simulink model "time"  (R2017b)
settings: Solver=FixedStepAuto  StartTime=0.0  StopTime=10.0  FixedStep=1  RelTol=1e-3
undefined symbols (not defined in the file): DiscIntNeverNeededParam
libraries: GPIO_Lib x6, TIMERS_Lib x3, USART_Lib x3, simulink x1
(part 1 of 2)
settings Model: Creator=edupc  LastModifiedBy=edupc

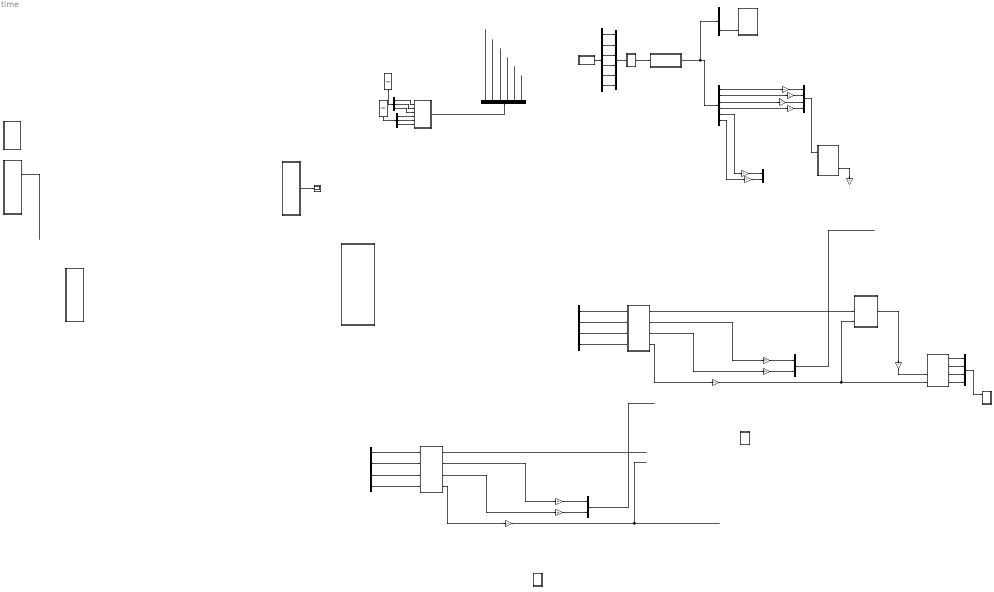
== system time ==
  Attitude : Subsystem  TreatAsAtomicUnit=on  SystemSampleTime=0.002
  Bus Creator : BusCreator  Inputs=6
  Bus Creator1 : BusCreator  Inputs=4
  Bus Creator2 : BusCreator  Inputs=2
  Bus Selector : BusSelector  OutputSignals=roll,pitch,yaw
  Bus Selector1 : BusSelector  OutputSignals=p,q,roll,pitch,yaw,r
  Chart : Stateflow chart  TreatAsAtomicUnit=on
  Chart1 : Stateflow chart  TreatAsAtomicUnit=on
  Chart2 : Stateflow chart  TreatAsAtomicUnit=on
  Chart3 : Stateflow chart  TreatAsAtomicUnit=on
  Chart4 : Stateflow chart  Priority=1  TreatAsAtomicUnit=on
  Chart9 : Stateflow chart  TreatAsAtomicUnit=on
  Data Type Conversion : DataTypeConversion  OutDataTypeStr=int32
  Data Type Conversion3 : DataTypeConversion  OutDataTypeStr=int32
  Demux1 : Demux
  Demux2 : Demux  Outputs=6
  Demux3 : Demux
  Demux4 : Demux  Outputs=3
  Demux5 : Demux  Outputs=3
  Demux6 : Demux  Outputs=6
  Filter : Subsystem  Tag=FilterWizardSubSystem  TreatAsAtomicUnit=on  SystemSampleTime=0.002
      settings: ErrorFcn=dspFilterRealizedInBasicElemsAlgLoopErrFcnCallback
  Gain{,1..2,11..13} (6 alike) : Gain  Gain=180/pi
  Gain10 : Gain  Gain=0.4
  Gain3 : Gain  Gain=30  ParamDataTypeStr=single
  Gain4 : Gain  Gain=30
  Gain5 : Gain  Gain=0.4
  Gain6 : Gain  Gain=-1  ParamDataTypeStr=single  OutDataTypeStr=single
  Gain7 : Gain  Gain=-1  ParamDataTypeStr=single  OutDataTypeStr=single
  Gain8 : Gain  Gain=30  ParamDataTypeStr=single
  Gain9 : Gain  Gain=30
  Mux1 : Mux  Inputs=2
  Mux2 : Mux
  Mux3 : Mux  Inputs=2
  PWM : Subsystem  TreatAsAtomicUnit=on
  Scope : Scope
  State Estimation and Complimentary Mixing : Subsystem  mask{EAComp=0.95}
      mask prompts: EAComp "Complimentary Filter Alpha:"
      mask TypeOptions EAComp: Complimentary Filter/EAComp
  Subsystem : Subsystem  TreatAsAtomicUnit=on  SystemSampleTime=0.002
  Subsystem1 : Subsystem  TreatAsAtomicUnit=on
  Subsystem5 : Subsystem  TreatAsAtomicUnit=on
  Yaw : Subsystem  TreatAsAtomicUnit=on  SystemSampleTime=0.002
  data scaling : Subsystem
  judgeLock : Subsystem  TreatAsAtomicUnit=on
  judgeLock1 : Subsystem  TreatAsAtomicUnit=on
  pwm_out1 : MATLAB Function  TreatAsAtomicUnit=on  SystemSampleTime=0.002
  wires:
  Chart/1(y) -> Scope/1
  Mux2/1 -> PWM/1(In1)
  Yaw/1(tau_yaw) -> Gain7/1
  Gain4/1 -> Mux1/2
  ? -> Yaw/1(states_estim)
  Gain5/1 -> Yaw/3(thrLow), pwm_out1/4(Thrust)
  Demux3/2 -> Subsystem5/2(pitchIn)
  Subsystem5/1(yaw) -> Yaw/2(yaw_ref)
  Subsystem5/4(thr) -> Gain5/1
  ? -> pwm_out1/2(Pitch)
  ? -> pwm_out1/1(Roll)
  Subsystem5/3(roll) -> Gain4/1
  pwm_out1/1(M1) -> Mux2/1
  Demux3/4 -> Subsystem5/4(yawIn)
  pwm_out1/3(M3) -> Mux2/3
  Demux3/3 -> Subsystem5/3(thrIn)
  Demux3/1 -> Subsystem5/1(rollIn)
  pwm_out1/2(M2) -> Mux2/2
  ? -> PWM/2(flyOk), judgeLock/1(In1)
  Subsystem5/2(pitch) -> Gain3/1
  Gain3/1 -> Mux1/1
  pwm_out1/4(M4) -> Mux2/4
  ? -> Demux3/1
  Gain7/1 -> pwm_out1/3(Yaw)
  Mux1/1 -> ?  "pitchRollCommand"
  Attitude/2(tau_pitch) -> Gain6/1
  Demux2/2 -> Bus Creator/2  "gy_filt"
  Bus Creator1/1 -> Attitude/1(states_estim)  "pitchRollBus"
  Bus Selector1/6 -> Gain13/1  "<r>"
  Bus Creator/1 -> data scaling/1(In1)
  Bus Selector1/2 -> Gain12/1  "<q>"
  Filter/1(Output) -> Demux2/1
  Demux2/6 -> Bus Creator/6  "az_filt"
  Bus Selector1/3 -> Gain/1  "<roll>"
  Demux2/1 -> Bus Creator/1  "gx_filt"
  Gain1/1 -> Bus Creator1/4  "pitch"
  Demux2/3 -> Bus Creator/3  "gz_filt"
  Gain12/1 -> Bus Creator1/2  "q"
  Bus Selector/3 -> Subsystem/3(yaw)  "<yaw>"
  Gain13/1 -> Bus Creator2/2  "r"
  Gain/1 -> Bus Creator1/3  "roll"
  Demux2/5 -> Bus Creator/5  "ay_filt"
  data scaling/1(Out1) -> State Estimation and Complimentary Mixing/1(In1)
  Gain11/1 -> Bus Creator1/1  "p"
  Bus Selector1/1 -> Gain11/1  "<p>"
  Bus Selector1/5 -> Gain2/1  "<yaw>"
  Gain2/1 -> Bus Creator2/1  "yaw"
  State Estimation and Complimentary Mixing/1(State Estimations) -> Bus Selector/1, Bus Selector1/1
  Demux2/4 -> Bus Creator/4  "ax_filt"
  Bus Selector1/4 -> Gain1/1  "<pitch>"
  ? -> ?  "input"
  Chart3/1(gyroData) -> ?
  Demux6/4 -> ?
  Demux4/3 -> Chart1/6(gz)
  Data Type Conversion3/1 -> Demux4/1
  Data Type Conversion/1 -> Demux5/1
  Demux6/2 -> ?
  Demux5/2 -> Chart1/2(ay)
  Demux4/2 -> Chart1/5(gy)
  Chart1/1(offset) -> Demux6/1
  Demux5/3 -> Chart1/3(az)
  Demux6/3 -> ?
  Demux6/1 -> ?
  Demux6/5 -> ?
  Demux4/1 -> Chart1/4(gx)
  Demux6/6 -> ?
  Demux5/1 -> Chart1/1(ax)
  ? -> Data Type Conversion3/1
  Demux1/2 -> Subsystem1/2(pitchIn)
  Demux1/4 -> Subsystem1/4(yawIn)
  Gain10/1 -> ?
  Demux1/1 -> Subsystem1/1(rollIn)
  Subsystem1/3(roll) -> Gain9/1
  Subsystem1/1(yaw) -> ?
  Gain9/1 -> Mux3/2
  ? -> judgeLock1/1(In1)
  Gain8/1 -> Mux3/1
  Subsystem1/4(thr) -> Gain10/1
  Subsystem1/2(pitch) -> Gain8/1
  Demux1/3 -> Subsystem1/3(thrIn)
  Mux3/1 -> ?  "pitchRollCommand"
  ? -> Demux1/1

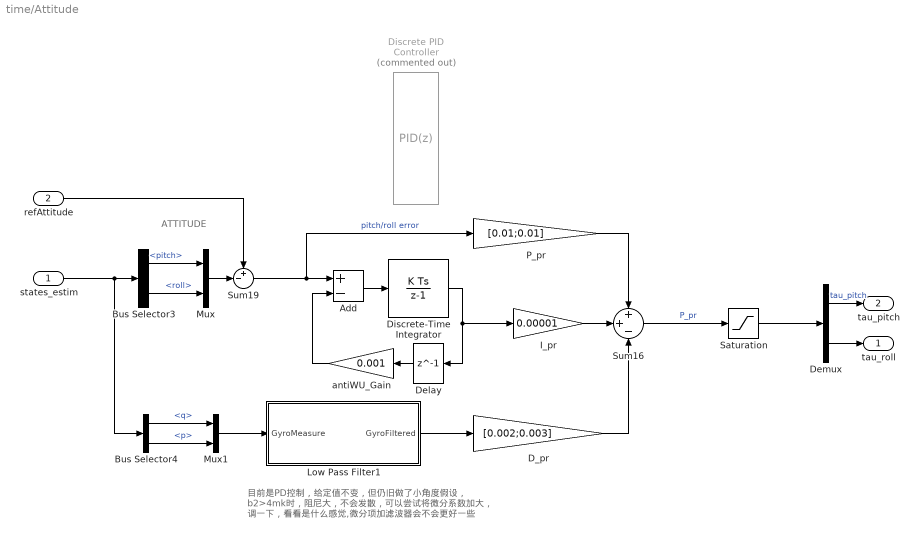
== system time/Attitude ==
  note: 目前是PD控制，给定值不变，但仍旧做了小角度假设，
      | b2>4mk时，阻尼大，不会发散，可以尝试将微分系数加大，
      | 调一下，看看是什么感觉,微分项加滤波器会不会更好一些
  note: ATTITUDE
  states_estim : Inport
  refAttitude : Inport  Port=2
  Add : Sum  Inputs=+-
  Bus Selector3 : BusSelector  OutputSignals=pitch,roll
  Bus Selector4 : BusSelector  OutputSignals=q,p
  D_pr : Gain  Gain=[0.002;0.003]  ParamDataTypeStr=single  OutDataTypeStr=single
  Delay : Delay  DelayLength=1  InitialCondition=0
  Demux : Demux  Outputs=2
  Discrete PID Controller : simulink/Continuous/PID Controller  Commented=on  Controller=PID  TimeDomain=Discrete-time  SampleTime=-1  IntegratorMethod=Forward Euler  FilterMethod=Forward Euler  Form=Parallel  UseFilter=on  ControllerParametersSource=external  P=1  I=1  D=0  N=100  InitialConditionSource=internal  InitialConditionForIntegrator=0  InitialConditionForFilter=0  ExternalReset=none  LimitOutput=off  UpperSaturationLimit=inf  LowerSaturationLimit=-inf  LinearizeAsGain=off  AntiWindupMode=none  Kb=1  TrackingMode=off  Kt=1  PParamMin=[]  PParamMax=[]  IParamMin=[]  IParamMax=[]  DParamMin=[]  DParamMax=[]  NParamMin=[]  NParamMax=[]  KbParamMin=[]  KbParamMax=[]  KtParamMin=[]  KtParamMax=[]  POutMin=[]  POutMax=[]  IOutMin=[]  IOutMax=[]  DOutMin=[]  DOutMax=[]  NOutMin=[]  NOutMax=[]  KbOutMin=[]  KbOutMax=[]  KtOutMin=[]  KtOutMax=[]  IntegratorOutMin=[]  IntegratorOutMax=[]  FilterOutMin=[]  FilterOutMax=[]  SumOutMin=[]  SumOutMax=[]  SumI1OutMin=[]  SumI1OutMax=[]  SumI2OutMin=[]  SumI2OutMax=[]  SumI3OutMin=[]  SumI3OutMax=[]  SumDOutMin=[]  SumDOutMax=[]  SaturationOutMin=[]  SaturationOutMax=[]  IntegratorContinuousStateAttributes=''  IntegratorStateMustResolveToSignalObject=off  IntegratorRTWStateStorageClass=Auto  FilterContinuousStateAttributes=''  FilterStateMustResolveToSignalObject=off  FilterRTWStateStorageClass=Auto  DifferentiatorICPrevScaledInput=0  DifferentiatorOutMin=[]  DifferentiatorOutMax=[]  InitialConditionSetting=State (most efficient)  FilterDiffOutCoefMin=[]  FilterDiffOutCoefMax=[]  SumDenOutMin=[]  SumDenOutMax=[]  SumNumOutMin=[]  SumNumOutMax=[]  ReciprocalOutMin=[]  ReciprocalOutMax=[]  DivideOutMin=[]  DivideOutMax=[]  TunerSelectOption=Transfer Function Based (PID Tuner App)
  Discrete-Time Integrator : DiscreteIntegrator  InitialConditionSetting=State (most efficient)  SampleTime=-1  LimitOutput=on  UpperSaturationLimit=0.1  LowerSaturationLimit=-0.1  ICPrevOutput=DiscIntNeverNeededParam  ICPrevScaledInput=DiscIntNeverNeededParam
  I_pr : Gain  Gain=0.00001  ParamDataTypeStr=single  OutDataTypeStr=single
  Low Pass Filter1 : Subsystem
  Mux : Mux  Inputs=2
  Mux1 : Mux  Inputs=2
  P_pr : Gain  Gain=[0.01;0.01]  ParamDataTypeStr=single  OutDataTypeStr=single
  Saturation : Saturate
  Sum16 : Sum  Inputs=++-  AccumDataTypeStr=single  OutDataTypeStr=single  SaturateOnIntegerOverflow=on
  Sum19 : Sum  Inputs=+-|
  antiWU_Gain : Gain  Gain=0.001
  tau_roll : Outport
  tau_pitch : Outport  Port=2
  wires:
  Mux1/1 -> Low Pass Filter1/1(GyroMeasure)
  Bus Selector4/2 -> Mux1/2  "<p>"
  Bus Selector3/2 -> Mux/2  "<roll>"
  Mux/1 -> Sum19/2
  refAttitude/1 -> Sum19/1
  states_estim/1 -> Bus Selector4/1, Bus Selector3/1
  D_pr/1 -> Sum16/3
  Demux/2 -> tau_roll/1
  Demux/1 -> tau_pitch/1  "tau_pitch"
  Delay/1 -> antiWU_Gain/1
  Discrete-Time Integrator/1 -> I_pr/1, Delay/1
  Sum19/1 -> P_pr/1, Add/1  "pitch/roll error"
  I_pr/1 -> Sum16/2
  P_pr/1 -> Sum16/1
  Bus Selector4/1 -> Mux1/1  "<q>"
  Bus Selector3/1 -> Mux/1  "<pitch>"
  Add/1 -> Discrete-Time Integrator/1
  antiWU_Gain/1 -> Add/2
  Sum16/1 -> Saturation/1  "P_pr"
  Saturation/1 -> Demux/1
  Low Pass Filter1/1(GyroFiltered) -> D_pr/1

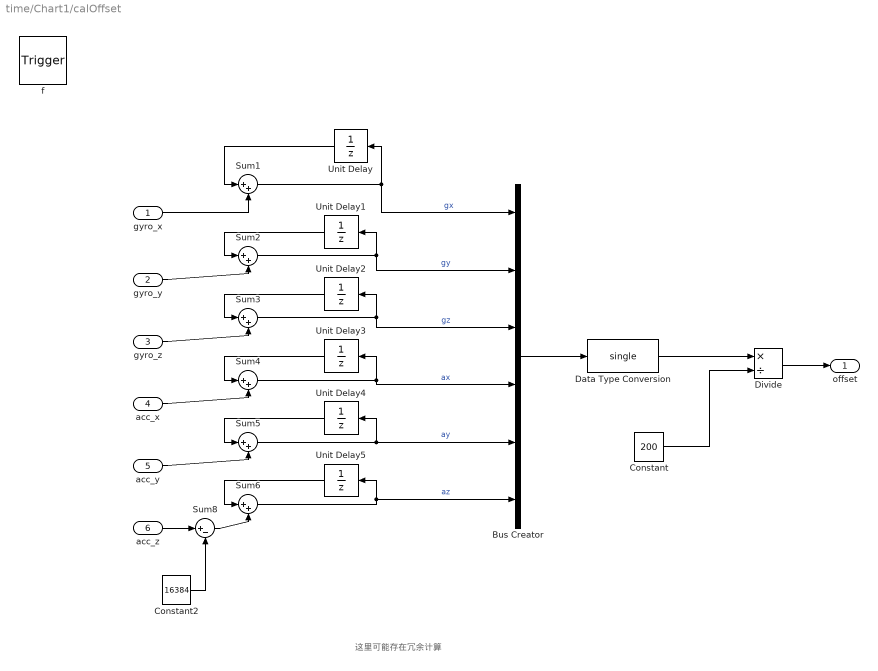
== system time/Chart1/calOffset ==
  note: 这里可能存在冗余计算
  gyro_x : Inport  OutDataTypeStr=int32
  gyro_y : Inport  Port=2  OutDataTypeStr=int32
  gyro_z : Inport  Port=3  OutDataTypeStr=int32
  acc_x : Inport  Port=4  OutDataTypeStr=int32
  acc_y : Inport  Port=5  OutDataTypeStr=int32
  acc_z : Inport  Port=6  OutDataTypeStr=int32
  f : TriggerPort  TriggerType=function-call  VariantControl=(inherit)
      settings: CopyFcn=Stateflow.SLINSF.SimulinkMan.removeBlockPreDeleteFcn  PreDeleteFcn=Stateflow.SLINSF.SimulinkMan.unsafePredeleteFcn
  Bus Creator : BusCreator  Inputs=6
  Constant : Constant  Value=200
  Constant2 : Constant  Value=16384  OutDataTypeStr=int16  SampleTime=-1
  Data Type Conversion : DataTypeConversion  OutDataTypeStr=single
  Divide : Product  Inputs=*/  OutDataTypeStr=single
  Sum{1..6} (6 alike) : Sum  Inputs=|++
  Sum8 : Sum  Inputs=|+-
  Unit Delay{,1..5} (6 alike) : UnitDelay  SampleTime=-1
  offset : Outport  OutDataTypeStr=single
  wires:
  gyro_x/1 -> Sum1/2
  Sum1/1 -> Bus Creator/1, Unit Delay/1  "gx"
  Unit Delay/1 -> Sum1/1
  gyro_y/1 -> Sum2/2
  Sum2/1 -> Unit Delay1/1, Bus Creator/2  "gy"
  Unit Delay1/1 -> Sum2/1
  Unit Delay2/1 -> Sum3/1
  Sum3/1 -> Unit Delay2/1, Bus Creator/3  "gz"
  Sum4/1 -> Unit Delay3/1, Bus Creator/4  "ax"
  Unit Delay3/1 -> Sum4/1
  Unit Delay4/1 -> Sum5/1
  Sum5/1 -> Unit Delay4/1, Bus Creator/5  "ay"
  Sum6/1 -> Bus Creator/6, Unit Delay5/1  "az"
  Unit Delay5/1 -> Sum6/1
  gyro_z/1 -> Sum3/2
  acc_x/1 -> Sum4/2
  acc_y/1 -> Sum5/2
  Bus Creator/1 -> Data Type Conversion/1
  acc_z/1 -> Sum8/1
  Sum8/1 -> Sum6/2
  Constant2/1 -> Sum8/2
  Constant/1 -> Divide/2
  Data Type Conversion/1 -> Divide/1
  Divide/1 -> offset/1

== system time/Chart4/pwmInit ==
  f : TriggerPort  TriggerType=function-call  VariantControl=(inherit)
      settings: CopyFcn=Stateflow.SLINSF.SimulinkMan.removeBlockPreDeleteFcn  PreDeleteFcn=Stateflow.SLINSF.SimulinkMan.unsafePredeleteFcn
  Constant : Constant
  Constant{10..13} (4 alike) : Constant  Value=0
  GPIO_Write : GPIO_Lib/GPIO_Write  Port_name=GPIOB  Pin0=off  Toggle_Pin0=off  Pin1=off  Toggle_Pin1=off  Pin2=on  Toggle_Pin2=off  Pin3=off  Toggle_Pin3=off  Pin4=off  Toggle_Pin4=off  Pin5=off  Toggle_Pin5=off  Pin6=off  Toggle_Pin6=off  Pin7=off  Toggle_Pin7=off  Pin8=off  Toggle_Pin8=off  Pin9=off  Toggle_Pin9=off  Pin10=off  Toggle_Pin10=off  Pin11=off  Toggle_Pin11=off  Pin12=off  Toggle_Pin12=off  Pin13=off  Toggle_Pin13=off  Pin14=off  Toggle_Pin14=off  Pin15=off  Toggle_Pin15=off  PinList="GPIOA4   8  11  12GPIOB1  2  3  6  7"
      settings: SourceProductName=Target Support Package - STM32 Adapter
  Timers : TIMERS_Lib/Timers  Priority=1  currentTIM=TIM2  TIM_Name=TIM2  TIM_APBClock=72000000  TIM_Set_Clk=on  TIM_Prescaler=71  TIM_Clock=1000000.00  Variable_frequency=off  TIM_Set_OutFreq=on  TIM_ARR=2500  Output_frequency=400.00  Repetition_counter=0  TIM_Mode=Up  TIM_DMA=none  TIM_IRQ=off  TIM_IRQ_ONLY=off  TIM_UP=off  TIM_TRG=off  TIM_COM=off  TIM_BRK=off  NbTIM=1  CH1_enable=on  CH1N_enable=off  CH1_type=Output_PWM  CH1_DMA=off  CH1_int=off  CH1_edge=Rising  CH1_div=1  CH1_variable_duty=on  CH1_set_pulse=off  CH1_output_duty=40.00  CH1_pulse=1000  CH2_enable=on  CH2N_enable=off  CH2_type=Output_PWM  CH2_DMA=off  CH2_int=off  CH2_edge=Rising  CH2_div=1  CH2_variable_duty=on  CH2_set_pulse=off  CH2_output_duty=40.00  CH2_pulse=1000  CH3_enable=on  CH3N_enable=off  CH3_type=Output_PWM  CH3_DMA=off  CH3_int=off  CH3_edge=Rising  CH3_div=1  CH3_variable_duty=on  CH3_set_pulse=off  CH3_output_duty=40.00  CH3_pulse=1000  CH4_enable=on  CH4N_enable=off  CH4_type=Output_PWM  CH4_DMA=off  CH4_int=off  CH4_edge=Rising  CH4_div=1  CH4_variable_duty=on  CH4_set_pulse=off  CH4_output_duty=40.00  CH4_pulse=1000
      settings: SourceProductName=Target Support Package - STM32 Adapter
  wires:
  Constant11/1 -> Timers/2
  Constant13/1 -> Timers/4
  Constant12/1 -> Timers/3
  Constant10/1 -> Timers/1
  Constant/1 -> GPIO_Write/1

== system time/Chart9/pwmInit ==
  f : TriggerPort  TriggerType=function-call  VariantControl=(inherit)
      settings: CopyFcn=Stateflow.SLINSF.SimulinkMan.removeBlockPreDeleteFcn  PreDeleteFcn=Stateflow.SLINSF.SimulinkMan.unsafePredeleteFcn
  Constant : Constant
  Constant{10..13} (4 alike) : Constant  Value=0
  GPIO_Write : GPIO_Lib/GPIO_Write  Port_name=GPIOB  Pin0=off  Toggle_Pin0=off  Pin1=off  Toggle_Pin1=off  Pin2=on  Toggle_Pin2=off  Pin3=off  Toggle_Pin3=off  Pin4=off  Toggle_Pin4=off  Pin5=off  Toggle_Pin5=off  Pin6=off  Toggle_Pin6=off  Pin7=off  Toggle_Pin7=off  Pin8=off  Toggle_Pin8=off  Pin9=off  Toggle_Pin9=off  Pin10=off  Toggle_Pin10=off  Pin11=off  Toggle_Pin11=off  Pin12=off  Toggle_Pin12=off  Pin13=off  Toggle_Pin13=off  Pin14=off  Toggle_Pin14=off  Pin15=off  Toggle_Pin15=off  PinList="GPIOA4   8  11  12GPIOB1  2  3  6  7"
      settings: SourceProductName=Target Support Package - STM32 Adapter
  Timers : TIMERS_Lib/Timers  Priority=1  currentTIM=TIM2  TIM_Name=TIM2  TIM_APBClock=72000000  TIM_Set_Clk=on  TIM_Prescaler=71  TIM_Clock=1000000.00  Variable_frequency=off  TIM_Set_OutFreq=on  TIM_ARR=2500  Output_frequency=400.00  Repetition_counter=0  TIM_Mode=Up  TIM_DMA=none  TIM_IRQ=off  TIM_IRQ_ONLY=off  TIM_UP=off  TIM_TRG=off  TIM_COM=off  TIM_BRK=off  NbTIM=1  CH1_enable=on  CH1N_enable=off  CH1_type=Output_PWM  CH1_DMA=off  CH1_int=off  CH1_edge=Rising  CH1_div=1  CH1_variable_duty=on  CH1_set_pulse=off  CH1_output_duty=40.00  CH1_pulse=1000  CH2_enable=on  CH2N_enable=off  CH2_type=Output_PWM  CH2_DMA=off  CH2_int=off  CH2_edge=Rising  CH2_div=1  CH2_variable_duty=on  CH2_set_pulse=off  CH2_output_duty=40.00  CH2_pulse=1000  CH3_enable=on  CH3N_enable=off  CH3_type=Output_PWM  CH3_DMA=off  CH3_int=off  CH3_edge=Rising  CH3_div=1  CH3_variable_duty=on  CH3_set_pulse=off  CH3_output_duty=40.00  CH3_pulse=1000  CH4_enable=on  CH4N_enable=off  CH4_type=Output_PWM  CH4_DMA=off  CH4_int=off  CH4_edge=Rising  CH4_div=1  CH4_variable_duty=on  CH4_set_pulse=off  CH4_output_duty=40.00  CH4_pulse=1000
      settings: SourceProductName=Target Support Package - STM32 Adapter
  wires:
  Constant11/1 -> Timers/2
  Constant13/1 -> Timers/4
  Constant12/1 -> Timers/3
  Constant10/1 -> Timers/1
  Constant/1 -> GPIO_Write/1

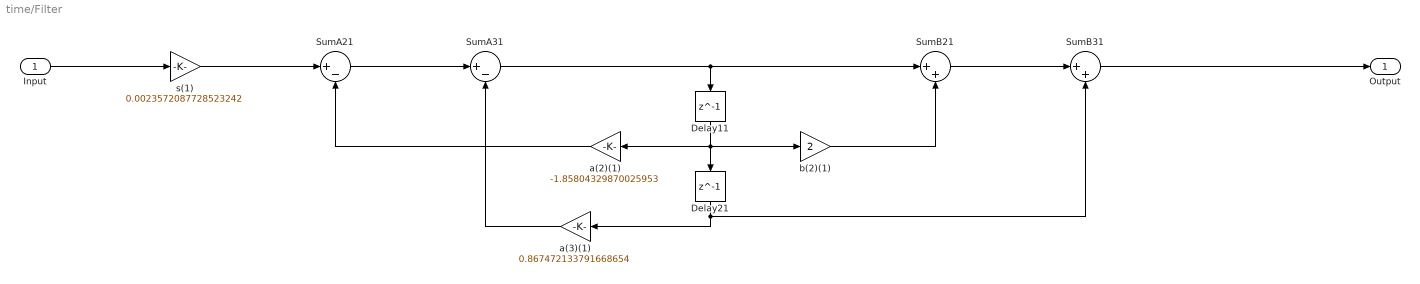
== system time/Filter ==
  Input : Inport
  Delay11 : Delay  DelayLength=1  InitialCondition=0
  Delay21 : Delay  DelayLength=1  InitialCondition=0
  SumA21 : Sum  Inputs=|+-  RndMeth=Nearest  SaturateOnIntegerOverflow=on  OutDataTypeStr=Inherit: Same as first input
  SumA31 : Sum  Inputs=|+-  RndMeth=Nearest  SaturateOnIntegerOverflow=on  OutDataTypeStr=Inherit: Same as first input
  SumB21 : Sum  Inputs=|++  RndMeth=Nearest  SaturateOnIntegerOverflow=on  OutDataTypeStr=Inherit: Same as first input
  SumB31 : Sum  Inputs=|++  RndMeth=Nearest  SaturateOnIntegerOverflow=on  OutDataTypeStr=Inherit: Same as first input
  a(2)(1) : Gain  Gain=-1.85804329870025953  ParamDataTypeStr=single  RndMeth=Nearest  SaturateOnIntegerOverflow=on  OutDataTypeStr=Inherit: Same as input
  a(3)(1) : Gain  Gain=0.867472133791668654  ParamDataTypeStr=single  RndMeth=Nearest  SaturateOnIntegerOverflow=on  OutDataTypeStr=Inherit: Same as input
  b(2)(1) : Gain  Gain=2  ParamDataTypeStr=single  RndMeth=Nearest  SaturateOnIntegerOverflow=on  OutDataTypeStr=Inherit: Same as input
  s(1) : Gain  Gain=0.0023572087728523242  ParamDataTypeStr=single  RndMeth=Nearest  SaturateOnIntegerOverflow=on  OutDataTypeStr=Inherit: Same as input
  Output : Outport
  wires:
  Input/1 -> s(1)/1
  s(1)/1 -> SumA21/1
  SumA21/1 -> SumA31/1
  SumA31/1 -> SumB21/1, Delay11/1
  SumB21/1 -> SumB31/1
  SumB31/1 -> Output/1
  a(2)(1)/1 -> SumA21/2
  Delay11/1 -> a(2)(1)/1, b(2)(1)/1, Delay21/1
  b(2)(1)/1 -> SumB21/2
  a(3)(1)/1 -> SumA31/2
  Delay21/1 -> a(3)(1)/1, SumB31/2

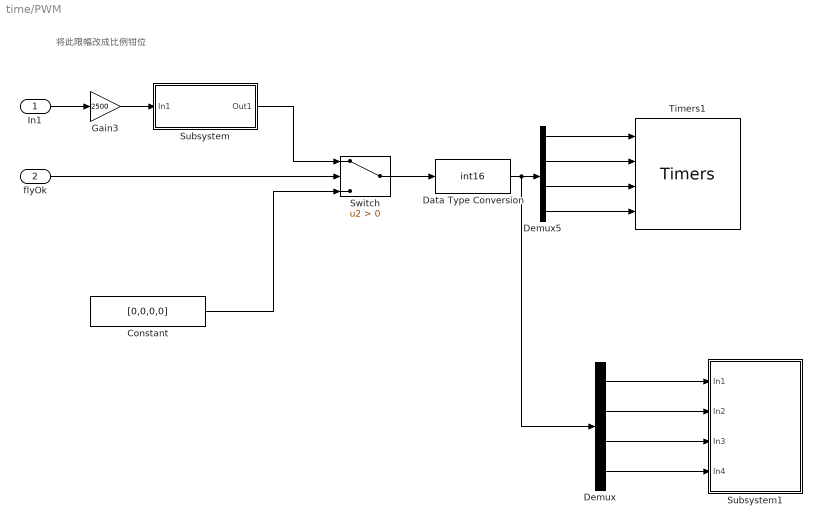
== system time/PWM ==
  note: 将此限幅改成比例钳位
  In1 : Inport
  flyOk : Inport  Port=2
  Constant : Constant  Value=[0,0,0,0]
  Data Type Conversion : DataTypeConversion  OutDataTypeStr=int16
  Demux : Demux
  Demux5 : Demux
  Gain3 : Gain  Gain=2500
  Subsystem : Subsystem
  Subsystem1 : Subsystem  TreatAsAtomicUnit=on
  Switch : Switch  Criteria=u2 > Threshold
  Timers1 : TIMERS_Lib/Timers  Priority=1  currentTIM=TIM2  TIM_Name=TIM2  TIM_APBClock=72000000  TIM_Set_Clk=on  TIM_Prescaler=71  TIM_Clock=1000000.00  Variable_frequency=off  TIM_Set_OutFreq=on  TIM_ARR=2500  Output_frequency=400.00  Repetition_counter=0  TIM_Mode=Up  TIM_DMA=none  TIM_IRQ=off  TIM_IRQ_ONLY=off  TIM_UP=off  TIM_TRG=off  TIM_COM=off  TIM_BRK=off  NbTIM=1  CH1_enable=on  CH1N_enable=off  CH1_type=Output_PWM  CH1_DMA=off  CH1_int=off  CH1_edge=Rising  CH1_div=1  CH1_variable_duty=on  CH1_set_pulse=off  CH1_output_duty=40.00  CH1_pulse=1000  CH2_enable=on  CH2N_enable=off  CH2_type=Output_PWM  CH2_DMA=off  CH2_int=off  CH2_edge=Rising  CH2_div=1  CH2_variable_duty=on  CH2_set_pulse=off  CH2_output_duty=40.00  CH2_pulse=1000  CH3_enable=on  CH3N_enable=off  CH3_type=Output_PWM  CH3_DMA=off  CH3_int=off  CH3_edge=Rising  CH3_div=1  CH3_variable_duty=on  CH3_set_pulse=off  CH3_output_duty=40.00  CH3_pulse=1000  CH4_enable=on  CH4N_enable=off  CH4_type=Output_PWM  CH4_DMA=off  CH4_int=off  CH4_edge=Rising  CH4_div=1  CH4_variable_duty=on  CH4_set_pulse=off  CH4_output_duty=40.00  CH4_pulse=1000
      settings: SourceProductName=Target Support Package - STM32 Adapter
  wires:
  Switch/1 -> Data Type Conversion/1
  Demux5/1 -> Timers1/1
  Demux5/4 -> Timers1/4
  Demux5/2 -> Timers1/2
  Demux5/3 -> Timers1/3
  flyOk/1 -> Switch/2
  Gain3/1 -> Subsystem/1(In1)
  In1/1 -> Gain3/1
  Data Type Conversion/1 -> Demux/1, Demux5/1
  Constant/1 -> Switch/3
  Subsystem/1(Out1) -> Switch/1
  Demux/1 -> Subsystem1/1(In1)
  Demux/2 -> Subsystem1/2(In2)
  Demux/3 -> Subsystem1/3(In3)
  Demux/4 -> Subsystem1/4(In4)

== system time/State Estimation and Complimentary Mixing ==
  note: The specific state estimation procedure employed in these bocks is
      | to be considered experimental (like everything else in this simulation).
      | While functional within the context of our application, this is not to be taken
      | as a "correct" method for state estimation or gyro/accelerometer data combination.
  note: Note:
      | x_gyro is taken as P,
      | y_gyro as Q,
      | z_gyro ad R.
  In1 : Inport
  Bus Creator : BusCreator  Inputs=6
  Bus Selector : BusSelector  OutputSignals=p,q,r,x_acc,y_acc,z_acc
  Complimentary Filter : Subsystem  mask{EAComp=EAComp}
      mask prompts: EAComp "Complimentary Filter Alpha:"
      mask TypeOptions EAComp: EAComp1/Gain
  Subsystem : Subsystem
  Subsystem1 : Subsystem
  State Estimations : Outport
  wires:
  In1/1 -> Bus Selector/1
  Bus Selector/1 -> Bus Creator/4, Subsystem/3(P)  "<p>"
  Bus Selector/3 -> Bus Creator/6, Subsystem/5(R)  "<r>"
  Bus Selector/2 -> Bus Creator/5, Subsystem/4(Q)  "<q>"
  Subsystem/2(thetaDot_gyro) -> Complimentary Filter/2(theDot_gyro)  "thateDot_gyro"
  Subsystem/3(psiDot_gyro) -> Complimentary Filter/3(psiDot_gyro)  "psiDot_gyro"
  Subsystem/1(phiDot_gyro) -> Complimentary Filter/1(phiDot_gyro)  "phiDot_gyro"
  Complimentary Filter/1(phi_est) -> Bus Creator/1, Subsystem/1(Phi)  "roll"
  Complimentary Filter/2(theta_est) -> Bus Creator/2, Subsystem/2(Theta)  "pitch"
  Complimentary Filter/3(psi_est) -> Bus Creator/3  "yaw"
  Subsystem1/2(phi_acc) -> Complimentary Filter/5(phiDot_acc)  "phi_acc"
  Subsystem1/1(theta_acc) -> Complimentary Filter/4(the_acc)  "theta_acc"
  Bus Selector/4 -> Subsystem1/1(x_acc)  "<x_acc>"
  Bus Selector/5 -> Subsystem1/2(y_acc)  "<y_acc>"
  Bus Selector/6 -> Subsystem1/3(z_acc)  "<z_acc>"
  Bus Creator/1 -> State Estimations/1

== system time/Subsystem ==
  roll : Inport
  pitch : Inport  Port=2
  yaw : Inport  Port=3
  Chart1 : Stateflow chart  TreatAsAtomicUnit=on
  wires:
  roll/1 -> Chart1/1(roll)
  yaw/1 -> Chart1/3(yaw)
  pitch/1 -> Chart1/2(pitch)

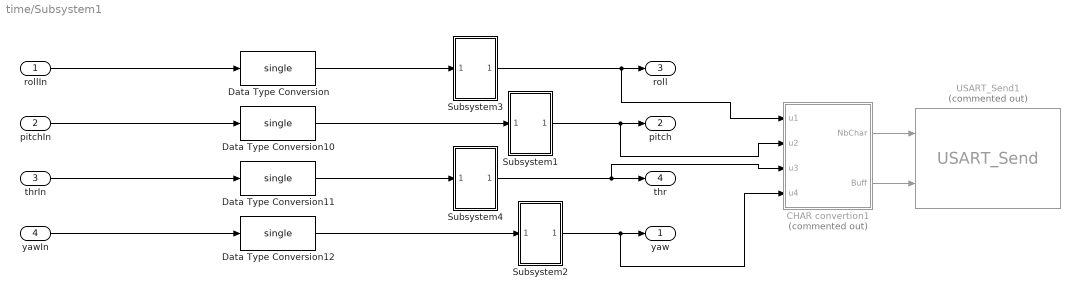
== system time/Subsystem1 ==
  rollIn : Inport
  pitchIn : Inport  Port=2
  thrIn : Inport  Port=3
  yawIn : Inport  Port=4
  CHAR convertion1 : MATLAB Function  Commented=on  TreatAsAtomicUnit=on
  Data Type Conversion{,10..12} (4 alike) : DataTypeConversion  OutDataTypeStr=single
  Subsystem1 : Subsystem
  Subsystem2 : Subsystem
  Subsystem3 : Subsystem
  Subsystem4 : Subsystem
  USART_Send1 : USART_Lib/USART_Send  Commented=on  USART_name=USART1  Buff_size=512  nbUsart=1  usartMode=Asynchronous  usartDma_Rx=off  usartDma_Tx=off  usartIt=on
      settings: SourceProductName=Target Support Package - STM32 Adapter
  yaw : Outport
  pitch : Outport  Port=2
  roll : Outport  Port=3
  thr : Outport  Port=4
  wires:
  Subsystem1/1(Out1) -> CHAR convertion1/2(u2), pitch/1
  Subsystem3/1(Out1) -> CHAR convertion1/1(u1), roll/1
  pitchIn/1 -> Data Type Conversion10/1
  yawIn/1 -> Data Type Conversion12/1
  rollIn/1 -> Data Type Conversion/1
  Data Type Conversion11/1 -> Subsystem4/1(In1)
  Data Type Conversion/1 -> Subsystem3/1(In1)
  Data Type Conversion12/1 -> Subsystem2/1(In1)
  Data Type Conversion10/1 -> Subsystem1/1(In1)
  thrIn/1 -> Data Type Conversion11/1
  Subsystem4/1(Out1) -> CHAR convertion1/3(u3), thr/1
  CHAR convertion1/2(Buff) -> USART_Send1/2
  CHAR convertion1/1(NbChar) -> USART_Send1/1
  Subsystem2/1(Out1) -> CHAR convertion1/4(u4), yaw/1

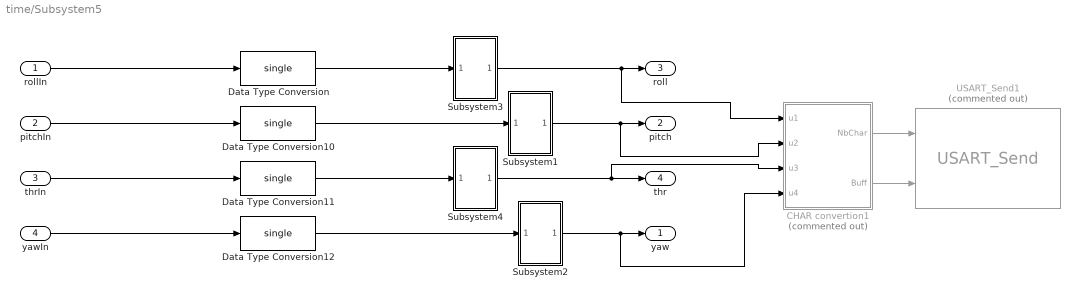
== system time/Subsystem5 ==
  rollIn : Inport
  pitchIn : Inport  Port=2
  thrIn : Inport  Port=3
  yawIn : Inport  Port=4
  CHAR convertion1 : MATLAB Function  Commented=on  TreatAsAtomicUnit=on
  Data Type Conversion{,10..12} (4 alike) : DataTypeConversion  OutDataTypeStr=single
  Subsystem1 : Subsystem
  Subsystem2 : Subsystem
  Subsystem3 : Subsystem
  Subsystem4 : Subsystem
  USART_Send1 : USART_Lib/USART_Send  Commented=on  USART_name=USART1  Buff_size=512  nbUsart=1  usartMode=Asynchronous  usartDma_Rx=off  usartDma_Tx=off  usartIt=on
      settings: SourceProductName=Target Support Package - STM32 Adapter
  yaw : Outport
  pitch : Outport  Port=2
  roll : Outport  Port=3
  thr : Outport  Port=4
  wires:
  Subsystem1/1(Out1) -> CHAR convertion1/2(u2), pitch/1
  Subsystem3/1(Out1) -> CHAR convertion1/1(u1), roll/1
  pitchIn/1 -> Data Type Conversion10/1
  yawIn/1 -> Data Type Conversion12/1
  rollIn/1 -> Data Type Conversion/1
  Data Type Conversion11/1 -> Subsystem4/1(In1)
  Data Type Conversion/1 -> Subsystem3/1(In1)
  Data Type Conversion12/1 -> Subsystem2/1(In1)
  Data Type Conversion10/1 -> Subsystem1/1(In1)
  thrIn/1 -> Data Type Conversion11/1
  Subsystem4/1(Out1) -> CHAR convertion1/3(u3), thr/1
  CHAR convertion1/2(Buff) -> USART_Send1/2
  CHAR convertion1/1(NbChar) -> USART_Send1/1
  Subsystem2/1(Out1) -> CHAR convertion1/4(u4), yaw/1

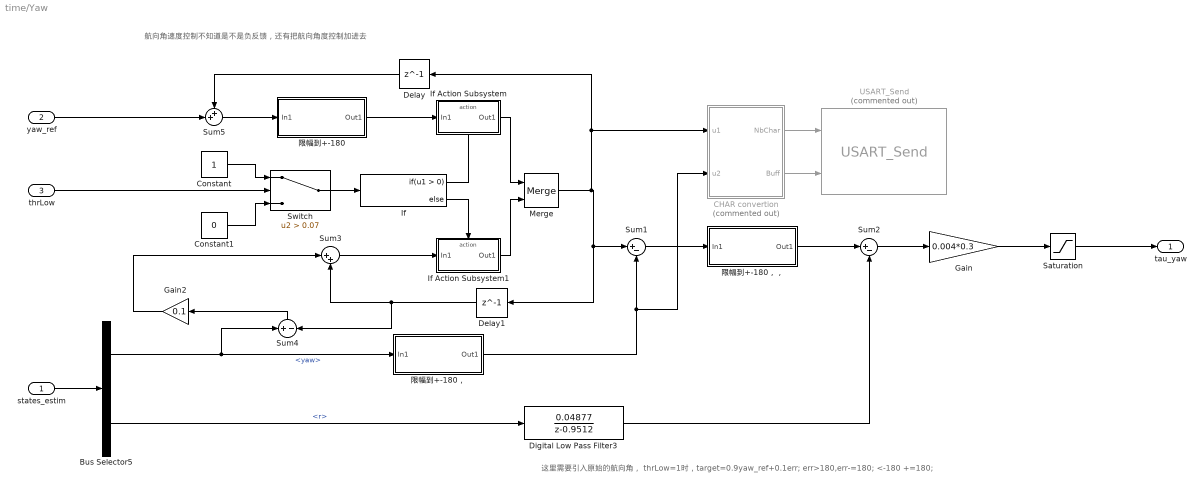
== system time/Yaw ==
  note: 这里需要引入原始的航向角，
      | thrLow=1时，target=0.9yaw_ref+0.1err;
      | err>180,err-=180;
      | <-180 +=180;
  note: 航向角速度控制不知道是不是负反馈，还有把航向角度控制加进去
  states_estim : Inport
  yaw_ref : Inport  Port=2
  thrLow : Inport  Port=3
  Bus Selector5 : BusSelector  OutputSignals=yaw,r
  CHAR convertion : MATLAB Function  Commented=on  TreatAsAtomicUnit=on
  Constant : Constant  OutDataTypeStr=int8
  Constant1 : Constant  Value=0  OutDataTypeStr=int8
  Delay : Delay  DelayLength=1
  Delay1 : Delay  DelayLength=1
  Digital Low Pass Filter3 : DiscreteTransferFcn  Numerator=[0.04877]  Denominator=[1 -0.9512]  OutDataTypeStr=int16
  Gain : Gain  Gain=0.004*0.3
  Gain2 : Gain  Gain=0.1
  If : If
  If Action Subsystem : Subsystem  TreatAsAtomicUnit=on
  If Action Subsystem1 : Subsystem  TreatAsAtomicUnit=on
  Merge : Merge
  Saturation : Saturate  UpperLimit=0.3  LowerLimit=-0.3
  Sum1 : Sum  Inputs=|+-
  Sum2 : Sum  Inputs=|+-
  Sum3 : Sum  Inputs=|++
  Sum4 : Sum  Inputs=+|-
  Sum5 : Sum  Inputs=++|
  Switch : Switch  Criteria=u2 > Threshold  Threshold=0.07
  USART_Send : USART_Lib/USART_Send  Commented=on  USART_name=USART1  Buff_size=512  nbUsart=1  usartMode=Asynchronous  usartDma_Rx=off  usartDma_Tx=off  usartIt=on
      settings: SourceProductName=Target Support Package - STM32 Adapter
  限幅到+-180 : Subsystem
  限幅到+-180， : Subsystem
  限幅到+-180，， : Subsystem
  tau_yaw : Outport
  wires:
  Gain/1 -> Saturation/1
  Sum2/1 -> Gain/1
  states_estim/1 -> Bus Selector5/1
  Bus Selector5/2 -> Digital Low Pass Filter3/1  "<r>"
  thrLow/1 -> Switch/2
  Constant/1 -> Switch/1
  Constant1/1 -> Switch/3
  Saturation/1 -> tau_yaw/1
  Switch/1 -> If/1
  If/1 -> If Action Subsystem/Action
  If Action Subsystem/1(Out1) -> Merge/1
  If/2 -> If Action Subsystem1/Action
  If Action Subsystem1/1(Out1) -> Merge/2
  Merge/1 -> CHAR convertion/1(u1), Delay/1, Delay1/1, Sum1/1
  Sum1/1 -> 限幅到+-180，，/1(In1)
  Bus Selector5/1 -> Sum4/1, 限幅到+-180，/1(In1)  "<yaw>"
  Sum3/1 -> If Action Subsystem1/1(In1)
  限幅到+-180/1(Out1) -> If Action Subsystem/1(In1)
  限幅到+-180，，/1(Out1) -> Sum2/1
  Sum5/1 -> 限幅到+-180/1(In1)
  yaw_ref/1 -> Sum5/2
  Delay/1 -> Sum5/1
  Delay1/1 -> Sum3/2, Sum4/2
  Sum4/1 -> Gain2/1
  Gain2/1 -> Sum3/1
  CHAR convertion/2(Buff) -> USART_Send/2
  CHAR convertion/1(NbChar) -> USART_Send/1
  限幅到+-180，/1(Out1) -> CHAR convertion/2(u2), Sum1/2
  Digital Low Pass Filter3/1 -> Sum2/2

== system time/data scaling ==
  note: For simulation, no
      | offset value is calculated.
  In1 : Inport
  Bus Creator : BusCreator  Inputs=6
  Bus Selector : BusSelector  OutputSignals=gx_filt,gy_filt,gz_filt,ax_filt,ay_filt,az_filt
  Demux : Demux  Outputs=3
  Demux1 : Demux  Outputs=3
  Gain : Gain  Gain=pi/(180*16.4)
  Gain1 : Gain  Gain=9.81/16384
  Mux1 : Mux  Inputs=3
  Mux2 : Mux  Inputs=3
  Out1 : Outport
  wires:
  In1/1 -> Bus Selector/1
  Bus Selector/1 -> Mux1/1  "<gx_filt>"
  Bus Selector/2 -> Mux1/2  "<gy_filt>"
  Bus Selector/3 -> Mux1/3  "<gz_filt>"
  Bus Selector/4 -> Mux2/1  "<ax_filt>"
  Bus Selector/5 -> Mux2/2  "<ay_filt>"
  Bus Selector/6 -> Mux2/3  "<az_filt>"
  Mux2/1 -> Gain1/1
  Mux1/1 -> Gain/1
  Gain1/1 -> Demux1/1
  Gain/1 -> Demux/1
  Demux/1 -> Bus Creator/1  "p"
  Demux/2 -> Bus Creator/2  "q"
  Demux/3 -> Bus Creator/3  "r"
  Demux1/1 -> Bus Creator/4  "x_acc"
  Demux1/2 -> Bus Creator/5  "y_acc"
  Demux1/3 -> Bus Creator/6  "z_acc"
  Bus Creator/1 -> Out1/1

== system time/judgeLock ==
  In1 : Inport
  Constant3 : Constant
  Constant4 : Constant  Value=0
  GPIO_Write : GPIO_Lib/GPIO_Write  Port_name=GPIOA  Pin0=off  Toggle_Pin0=off  Pin1=off  Toggle_Pin1=off  Pin2=off  Toggle_Pin2=off  Pin3=off  Toggle_Pin3=off  Pin4=off  Toggle_Pin4=off  Pin5=off  Toggle_Pin5=off  Pin6=off  Toggle_Pin6=off  Pin7=off  Toggle_Pin7=off  Pin8=on  Toggle_Pin8=off  Pin9=off  Toggle_Pin9=off  Pin10=off  Toggle_Pin10=off  Pin11=on  Toggle_Pin11=off  Pin12=off  Toggle_Pin12=off  Pin13=off  Toggle_Pin13=off  Pin14=off  Toggle_Pin14=off  Pin15=off  Toggle_Pin15=off  PinList="GPIOA4   8  11  12GPIOB1  2  3  6  7"
      settings: SourceProductName=Target Support Package - STM32 Adapter
  GPIO_Write1 : GPIO_Lib/GPIO_Write  Port_name=GPIOB  Pin0=off  Toggle_Pin0=off  Pin1=on  Toggle_Pin1=off  Pin2=off  Toggle_Pin2=off  Pin3=on  Toggle_Pin3=off  Pin4=off  Toggle_Pin4=off  Pin5=off  Toggle_Pin5=off  Pin6=off  Toggle_Pin6=off  Pin7=off  Toggle_Pin7=off  Pin8=off  Toggle_Pin8=off  Pin9=off  Toggle_Pin9=off  Pin10=off  Toggle_Pin10=off  Pin11=off  Toggle_Pin11=off  Pin12=off  Toggle_Pin12=off  Pin13=off  Toggle_Pin13=off  Pin14=off  Toggle_Pin14=off  Pin15=off  Toggle_Pin15=off  PinList="GPIOA4   8  11  12GPIOB1  2  3  6  7"
      settings: SourceProductName=Target Support Package - STM32 Adapter
  If : If
  If Action Subsystem : Subsystem  TreatAsAtomicUnit=on
  If Action Subsystem1 : Subsystem  TreatAsAtomicUnit=on
  Merge : Merge
  wires:
  In1/1 -> If/1
  Constant4/1 -> If Action Subsystem1/1(In1)
  Constant3/1 -> If Action Subsystem/1(In1)
  If Action Subsystem1/1(Out1) -> Merge/2
  If/1 -> If Action Subsystem/Action
  If/2 -> If Action Subsystem1/Action
  If Action Subsystem/1(Out1) -> Merge/1
  Merge/1 -> GPIO_Write/1, GPIO_Write/2, GPIO_Write1/2, GPIO_Write1/1

== system time/judgeLock1 ==
  In1 : Inport
  Constant3 : Constant
  Constant4 : Constant  Value=0
  GPIO_Write : GPIO_Lib/GPIO_Write  Port_name=GPIOA  Pin0=off  Toggle_Pin0=off  Pin1=off  Toggle_Pin1=off  Pin2=off  Toggle_Pin2=off  Pin3=off  Toggle_Pin3=off  Pin4=off  Toggle_Pin4=off  Pin5=off  Toggle_Pin5=off  Pin6=off  Toggle_Pin6=off  Pin7=off  Toggle_Pin7=off  Pin8=on  Toggle_Pin8=off  Pin9=off  Toggle_Pin9=off  Pin10=off  Toggle_Pin10=off  Pin11=on  Toggle_Pin11=off  Pin12=off  Toggle_Pin12=off  Pin13=off  Toggle_Pin13=off  Pin14=off  Toggle_Pin14=off  Pin15=off  Toggle_Pin15=off  PinList="GPIOA4   8  11  12GPIOB1  2  3  6  7"
      settings: SourceProductName=Target Support Package - STM32 Adapter
  GPIO_Write1 : GPIO_Lib/GPIO_Write  Port_name=GPIOB  Pin0=off  Toggle_Pin0=off  Pin1=on  Toggle_Pin1=off  Pin2=off  Toggle_Pin2=off  Pin3=on  Toggle_Pin3=off  Pin4=off  Toggle_Pin4=off  Pin5=off  Toggle_Pin5=off  Pin6=off  Toggle_Pin6=off  Pin7=off  Toggle_Pin7=off  Pin8=off  Toggle_Pin8=off  Pin9=off  Toggle_Pin9=off  Pin10=off  Toggle_Pin10=off  Pin11=off  Toggle_Pin11=off  Pin12=off  Toggle_Pin12=off  Pin13=off  Toggle_Pin13=off  Pin14=off  Toggle_Pin14=off  Pin15=off  Toggle_Pin15=off  PinList="GPIOA4   8  11  12GPIOB1  2  3  6  7"
      settings: SourceProductName=Target Support Package - STM32 Adapter
  If : If
  If Action Subsystem : Subsystem  TreatAsAtomicUnit=on
  If Action Subsystem1 : Subsystem  TreatAsAtomicUnit=on
  Merge : Merge
  wires:
  In1/1 -> If/1
  Constant4/1 -> If Action Subsystem1/1(In1)
  Constant3/1 -> If Action Subsystem/1(In1)
  If Action Subsystem1/1(Out1) -> Merge/2
  If/1 -> If Action Subsystem/Action
  If/2 -> If Action Subsystem1/Action
  If Action Subsystem/1(Out1) -> Merge/1
  Merge/1 -> GPIO_Write/1, GPIO_Write/2, GPIO_Write1/2, GPIO_Write1/1

== system time/Attitude/Low Pass Filter1 ==
  GyroMeasure : Inport
  Demux : Demux  Outputs=2
  Digital Low Pass Filter1 : DiscreteTransferFcn  Numerator=[0.04877]  Denominator=[1 -0.9512]  OutDataTypeStr=int16
  Digital Low Pass Filter2 : DiscreteTransferFcn  Numerator=[0.04877]  Denominator=[1 -0.9512]  OutDataTypeStr=int16
  Mux3 : Mux  Inputs=2
  GyroFiltered : Outport
  wires:
  Mux3/1 -> GyroFiltered/1
  Demux/1 -> Digital Low Pass Filter2/1
  GyroMeasure/1 -> Demux/1
  Demux/2 -> Digital Low Pass Filter1/1
  Digital Low Pass Filter2/1 -> Mux3/1
  Digital Low Pass Filter1/1 -> Mux3/2

== system time/PWM/Subsystem ==
  In1 : Inport
  Demux : Demux
  Divide : Product  Inputs=*/
  Gain : Gain  Gain=1200
  If : If  IfExpression=u1 > 1200
  If Action Subsystem : Subsystem  TreatAsAtomicUnit=on
  If Action Subsystem1 : Subsystem  TreatAsAtomicUnit=on
  Merge : Merge
  Min : MinMax  Function=max  Inputs=4
  Out1 : Outport
  wires:
  Demux/4 -> Min/4
  In1/1 -> Divide/1, If Action Subsystem1/1(In1), Demux/1
  Demux/1 -> Min/1
  Demux/2 -> Min/2
  Demux/3 -> Min/3
  If/1 -> If Action Subsystem/Action
  If/2 -> If Action Subsystem1/Action
  If Action Subsystem/1(Out1) -> Merge/1
  If Action Subsystem1/1(Out1) -> Merge/2
  Min/1 -> Divide/2, If/1
  Gain/1 -> If Action Subsystem/1(In1)
  Divide/1 -> Gain/1
  Merge/1 -> Out1/1

== system time/PWM/Subsystem1 ==
  In1 : Inport
  In2 : Inport  Port=2
  In3 : Inport  Port=3
  In4 : Inport  Port=4
  Chart1 : Stateflow chart  TreatAsAtomicUnit=on
  wires:
  In1/1 -> Chart1/1(m_1)
  In2/1 -> Chart1/2(m_2)
  In3/1 -> Chart1/3(m_3)
  In4/1 -> Chart1/4(m_4)

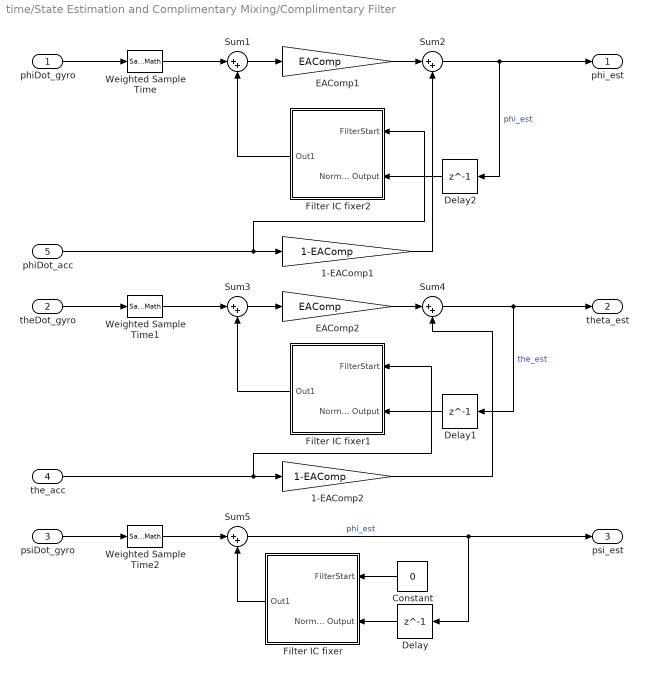
== system time/State Estimation and Complimentary Mixing/Complimentary Filter ==
  phiDot_gyro : Inport
  theDot_gyro : Inport  Port=2
  psiDot_gyro : Inport  Port=3
  the_acc : Inport  Port=4
  phiDot_acc : Inport  Port=5
  1-EAComp1 : Gain  Gain=1-EAComp
  1-EAComp2 : Gain  Gain=1-EAComp
  Constant : Constant  Value=0  OutDataTypeStr=single
  Delay : Delay  DelayLength=1  InitialCondition=0
  Delay1 : Delay  DelayLength=1  InitialCondition=0
  Delay2 : Delay  DelayLength=1  InitialCondition=0
  EAComp1 : Gain  Gain=EAComp
  EAComp2 : Gain  Gain=EAComp
  Filter IC fixer : Subsystem
  Filter IC fixer1 : Subsystem
  Filter IC fixer2 : Subsystem
  Sum{1..4} (4 alike) : Sum  Inputs=|++
  Sum5 : Sum  Inputs=|++  OutDataTypeStr=single
  Weighted Sample Time : SampleTimeMath  TsampMathOp=*
  Weighted Sample Time1 : SampleTimeMath  TsampMathOp=*
  Weighted Sample Time2 : SampleTimeMath  TsampMathOp=*
  phi_est : Outport
  theta_est : Outport  Port=2
  psi_est : Outport  Port=3  OutDataTypeStr=single
  wires:
  Weighted Sample Time/1 -> Sum1/1
  Sum1/1 -> EAComp1/1
  Sum2/1 -> Delay2/1, phi_est/1  "phi_est"
  1-EAComp1/1 -> Sum2/2
  phiDot_gyro/1 -> Weighted Sample Time/1
  phiDot_acc/1 -> Filter IC fixer2/1(FilterStart), 1-EAComp1/1
  EAComp1/1 -> Sum2/1
  Weighted Sample Time1/1 -> Sum3/1
  Sum3/1 -> EAComp2/1
  Sum4/1 -> Delay1/1, theta_est/1  "the_est"
  1-EAComp2/1 -> Sum4/2
  theDot_gyro/1 -> Weighted Sample Time1/1
  the_acc/1 -> 1-EAComp2/1, Filter IC fixer1/1(FilterStart)
  EAComp2/1 -> Sum4/1
  psiDot_gyro/1 -> Weighted Sample Time2/1
  Weighted Sample Time2/1 -> Sum5/1
  Sum5/1 -> Delay/1, psi_est/1  "phi_est"
  Delay/1 -> Filter IC fixer/2(Normal Output)
  Filter IC fixer/1(Out1) -> Sum5/2
  Constant/1 -> Filter IC fixer/1(FilterStart)
  Filter IC fixer1/1(Out1) -> Sum3/2
  Filter IC fixer2/1(Out1) -> Sum1/2
  Delay1/1 -> Filter IC fixer1/2(Normal Output)
  Delay2/1 -> Filter IC fixer2/2(Normal Output)

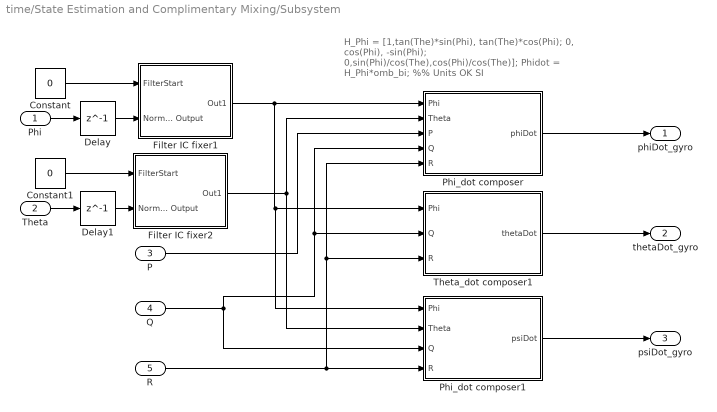
== system time/State Estimation and Complimentary Mixing/Subsystem ==
  note: H_Phi = [1,tan(The)*sin(Phi), tan(The)*cos(Phi);
      |          0,         cos(Phi),         -sin(Phi);
      |          0,sin(Phi)/cos(The),cos(Phi)/cos(The)];
      | Phidot = H_Phi*omb_bi; %% Units OK SI
  Phi : Inport  OutDataTypeStr=single
  Theta : Inport  Port=2
  P : Inport  Port=3
  Q : Inport  Port=4
  R : Inport  Port=5
  Constant : Constant  Value=0  OutDataTypeStr=single
  Constant1 : Constant  Value=0  OutDataTypeStr=single
  Delay : Delay  DelayLength=1  InitialCondition=0
  Delay1 : Delay  DelayLength=1  InitialCondition=0
  Filter IC fixer1 : Subsystem
  Filter IC fixer2 : Subsystem
  Phi_dot composer : Subsystem
  Phi_dot composer1 : Subsystem
  Theta_dot composer1 : Subsystem
  phiDot_gyro : Outport
  thetaDot_gyro : Outport  Port=2
  psiDot_gyro : Outport  Port=3
  wires:
  P/1 -> Phi_dot composer/3(P)
  Q/1 -> Phi_dot composer1/3(Q), Theta_dot composer1/2(Q), Phi_dot composer/4(Q)
  Phi_dot composer/1(phiDot) -> phiDot_gyro/1
  Theta_dot composer1/1(thetaDot) -> thetaDot_gyro/1
  R/1 -> Theta_dot composer1/3(R), Phi_dot composer/5(R), Phi_dot composer1/4(R)
  Phi_dot composer1/1(psiDot) -> psiDot_gyro/1
  Filter IC fixer1/1(Out1) -> Phi_dot composer1/1(Phi), Theta_dot composer1/1(Phi), Phi_dot composer/1(Phi)
  Delay/1 -> Filter IC fixer1/2(Normal Output)
  Phi/1 -> Delay/1
  Constant/1 -> Filter IC fixer1/1(FilterStart)
  Theta/1 -> Delay1/1
  Filter IC fixer2/1(Out1) -> Phi_dot composer/2(Theta), Phi_dot composer1/2(Theta)
  Delay1/1 -> Filter IC fixer2/2(Normal Output)
  Constant1/1 -> Filter IC fixer2/1(FilterStart)

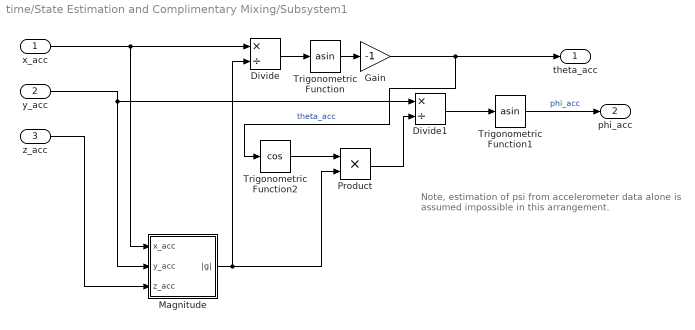
== system time/State Estimation and Complimentary Mixing/Subsystem1 ==
  note: Note, estimation of psi from accelerometer data alone
      | is assumed impossible in this arrangement.
  x_acc : Inport
  y_acc : Inport  Port=2
  z_acc : Inport  Port=3
  Divide : Product  Inputs=*/
  Divide1 : Product  Inputs=*/
  Gain : Gain  Gain=-1
  Magnitude : Subsystem
  Product : Product
  Trigonometric Function : Trigonometry  Operator=asin  OutputSignalType=real
  Trigonometric Function1 : Trigonometry  Operator=asin  OutputSignalType=real
  Trigonometric Function2 : Trigonometry  Operator=cos  OutputSignalType=real
  theta_acc : Outport
  phi_acc : Outport  Port=2
  wires:
  Divide/1 -> Trigonometric Function/1
  Magnitude/1(|g|) -> Product/2, Divide/2
  Trigonometric Function2/1 -> Product/1
  Trigonometric Function/1 -> Gain/1
  y_acc/1 -> Magnitude/2(y_acc), Divide1/1
  z_acc/1 -> Magnitude/3(z_acc)
  Divide1/1 -> Trigonometric Function1/1
  Product/1 -> Divide1/2
  Trigonometric Function1/1 -> phi_acc/1  "phi_acc"
  x_acc/1 -> Magnitude/1(x_acc), Divide/1
  Gain/1 -> theta_acc/1, Trigonometric Function2/1  "theta_acc"

== system time/Subsystem1/Subsystem1 ==
  In1 : Inport
  Constant3 : Constant  Value=1500  OutDataTypeStr=single
  Constant4 : Constant  Value=500  OutDataTypeStr=single
  Dead Zone : DeadZone  LowerValue=-85  UpperValue=85  SaturateOnIntegerOverflow=on
  Divide1 : Product  Inputs=*/
  Saturation4 : Saturate  UpperLimit=2000  LowerLimit=1000
  Sum1 : Sum  Inputs=|+-
  Out1 : Outport
  wires:
  Divide1/1 -> Out1/1
  Dead Zone/1 -> Divide1/1
  Constant3/1 -> Sum1/2
  Saturation4/1 -> Sum1/1
  Constant4/1 -> Divide1/2
  In1/1 -> Saturation4/1
  Sum1/1 -> Dead Zone/1

== system time/Subsystem1/Subsystem2 ==
  In1 : Inport
  Constant3 : Constant  Value=1500  OutDataTypeStr=single
  Constant4 : Constant  Value=500  OutDataTypeStr=single
  Dead Zone : DeadZone  LowerValue=-85  UpperValue=85  SaturateOnIntegerOverflow=on
  Divide1 : Product  Inputs=*/
  Saturation4 : Saturate  UpperLimit=2000  LowerLimit=1000
  Sum1 : Sum  Inputs=|+-
  Out1 : Outport
  wires:
  Sum1/1 -> Dead Zone/1
  In1/1 -> Saturation4/1
  Constant4/1 -> Divide1/2
  Saturation4/1 -> Sum1/1
  Constant3/1 -> Sum1/2
  Dead Zone/1 -> Divide1/1
  Divide1/1 -> Out1/1

== system time/Subsystem1/Subsystem3 ==
  In1 : Inport
  Constant3 : Constant  Value=1500  OutDataTypeStr=single
  Constant4 : Constant  Value=500  OutDataTypeStr=single
  Dead Zone : DeadZone  LowerValue=-85  UpperValue=85  SaturateOnIntegerOverflow=on
  Divide1 : Product  Inputs=*/
  Saturation4 : Saturate  UpperLimit=2000  LowerLimit=1000
  Sum1 : Sum  Inputs=|+-
  Out1 : Outport
  wires:
  Sum1/1 -> Dead Zone/1
  In1/1 -> Saturation4/1
  Constant4/1 -> Divide1/2
  Saturation4/1 -> Sum1/1
  Constant3/1 -> Sum1/2
  Dead Zone/1 -> Divide1/1
  Divide1/1 -> Out1/1

== system time/Subsystem1/Subsystem4 ==
  In1 : Inport
  Constant3 : Constant  Value=1000  OutDataTypeStr=single
  Constant4 : Constant  Value=1000  OutDataTypeStr=single
  Divide1 : Product  Inputs=*/
  Saturation4 : Saturate  UpperLimit=2000  LowerLimit=1000
  Sum1 : Sum  Inputs=|+-
  Out1 : Outport
  wires:
  Divide1/1 -> Out1/1
  Sum1/1 -> Divide1/1
  Constant3/1 -> Sum1/2
  Saturation4/1 -> Sum1/1
  Constant4/1 -> Divide1/2
  In1/1 -> Saturation4/1

== system time/Subsystem5/Subsystem1 ==
  In1 : Inport
  Constant3 : Constant  Value=1500  OutDataTypeStr=single
  Constant4 : Constant  Value=500  OutDataTypeStr=single
  Dead Zone : DeadZone  LowerValue=-85  UpperValue=85  SaturateOnIntegerOverflow=on
  Divide1 : Product  Inputs=*/
  Saturation4 : Saturate  UpperLimit=2000  LowerLimit=1000
  Sum1 : Sum  Inputs=|+-
  Out1 : Outport
  wires:
  Divide1/1 -> Out1/1
  Dead Zone/1 -> Divide1/1
  Constant3/1 -> Sum1/2
  Saturation4/1 -> Sum1/1
  Constant4/1 -> Divide1/2
  In1/1 -> Saturation4/1
  Sum1/1 -> Dead Zone/1

== system time/Subsystem5/Subsystem2 ==
  In1 : Inport
  Constant3 : Constant  Value=1500  OutDataTypeStr=single
  Constant4 : Constant  Value=500  OutDataTypeStr=single
  Dead Zone : DeadZone  LowerValue=-85  UpperValue=85  SaturateOnIntegerOverflow=on
  Divide1 : Product  Inputs=*/
  Saturation4 : Saturate  UpperLimit=2000  LowerLimit=1000
  Sum1 : Sum  Inputs=|+-
  Out1 : Outport
  wires:
  Sum1/1 -> Dead Zone/1
  In1/1 -> Saturation4/1
  Constant4/1 -> Divide1/2
  Saturation4/1 -> Sum1/1
  Constant3/1 -> Sum1/2
  Dead Zone/1 -> Divide1/1
  Divide1/1 -> Out1/1

== system time/Subsystem5/Subsystem3 ==
  In1 : Inport
  Constant3 : Constant  Value=1500  OutDataTypeStr=single
  Constant4 : Constant  Value=500  OutDataTypeStr=single
  Dead Zone : DeadZone  LowerValue=-85  UpperValue=85  SaturateOnIntegerOverflow=on
  Divide1 : Product  Inputs=*/
  Saturation4 : Saturate  UpperLimit=2000  LowerLimit=1000
  Sum1 : Sum  Inputs=|+-
  Out1 : Outport
  wires:
  Sum1/1 -> Dead Zone/1
  In1/1 -> Saturation4/1
  Constant4/1 -> Divide1/2
  Saturation4/1 -> Sum1/1
  Constant3/1 -> Sum1/2
  Dead Zone/1 -> Divide1/1
  Divide1/1 -> Out1/1

== system time/Subsystem5/Subsystem4 ==
  In1 : Inport
  Constant3 : Constant  Value=1000  OutDataTypeStr=single
  Constant4 : Constant  Value=1000  OutDataTypeStr=single
  Divide1 : Product  Inputs=*/
  Saturation4 : Saturate  UpperLimit=2000  LowerLimit=1000
  Sum1 : Sum  Inputs=|+-
  Out1 : Outport
  wires:
  Divide1/1 -> Out1/1
  Sum1/1 -> Divide1/1
  Constant3/1 -> Sum1/2
  Saturation4/1 -> Sum1/1
  Constant4/1 -> Divide1/2
  In1/1 -> Saturation4/1

== system time/Yaw/If Action Subsystem ==
  In1 : Inport
  Action Port : ActionPort
  Out1 : Outport
  wires:
  In1/1 -> Out1/1

== system time/Yaw/If Action Subsystem1 ==
  In1 : Inport
  Action Port : ActionPort
  Out1 : Outport
  wires:
  In1/1 -> Out1/1

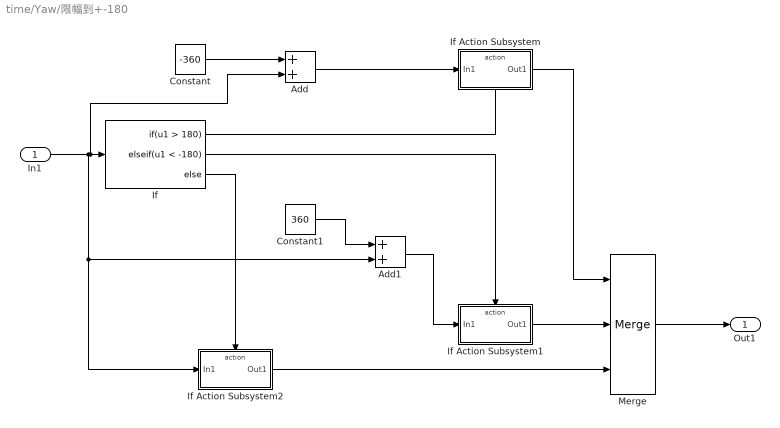
== system time/Yaw/限幅到+-180 ==
  In1 : Inport  OutDataTypeStr=single
  Add : Sum
  Add1 : Sum
  Constant : Constant  Value=-360  OutDataTypeStr=single
  Constant1 : Constant  Value=360  OutDataTypeStr=single
  If : If  IfExpression=u1 > 180  ElseIfExpressions=u1 < -180
  If Action Subsystem : Subsystem  TreatAsAtomicUnit=on
  If Action Subsystem1 : Subsystem  TreatAsAtomicUnit=on
  If Action Subsystem2 : Subsystem  TreatAsAtomicUnit=on
  Merge : Merge  Inputs=3
  Out1 : Outport
  wires:
  In1/1 -> Add1/2, If Action Subsystem2/1(In1), Add/2, If/1
  If/1 -> If Action Subsystem/Action
  If/2 -> If Action Subsystem1/Action
  If/3 -> If Action Subsystem2/Action
  If Action Subsystem/1(Out1) -> Merge/1
  Constant/1 -> Add/1
  Add/1 -> If Action Subsystem/1(In1)
  If Action Subsystem1/1(Out1) -> Merge/2
  Constant1/1 -> Add1/1
  If Action Subsystem2/1(Out1) -> Merge/3
  Add1/1 -> If Action Subsystem1/1(In1)
  Merge/1 -> Out1/1

== system time/Yaw/限幅到+-180， ==
  In1 : Inport  OutDataTypeStr=single
  Add : Sum
  Add1 : Sum
  Constant : Constant  Value=-360  OutDataTypeStr=single
  Constant1 : Constant  Value=360  OutDataTypeStr=single
  If : If  IfExpression=u1 > 180  ElseIfExpressions=u1 < -180
  If Action Subsystem : Subsystem  TreatAsAtomicUnit=on
  If Action Subsystem1 : Subsystem  TreatAsAtomicUnit=on
  If Action Subsystem2 : Subsystem  TreatAsAtomicUnit=on
  Merge : Merge  Inputs=3
  Out1 : Outport
  wires:
  Merge/1 -> Out1/1
  Add1/1 -> If Action Subsystem1/1(In1)
  If Action Subsystem2/1(Out1) -> Merge/3
  Constant1/1 -> Add1/1
  If Action Subsystem1/1(Out1) -> Merge/2
  Add/1 -> If Action Subsystem/1(In1)
  Constant/1 -> Add/1
  If Action Subsystem/1(Out1) -> Merge/1
  If/3 -> If Action Subsystem2/Action
  If/2 -> If Action Subsystem1/Action
  If/1 -> If Action Subsystem/Action
  In1/1 -> If/1, Add/2, If Action Subsystem2/1(In1), Add1/2

== system time/Yaw/限幅到+-180，， ==
  In1 : Inport  OutDataTypeStr=single
  Add : Sum
  Add1 : Sum
  Constant : Constant  Value=-360  OutDataTypeStr=single
  Constant1 : Constant  Value=360  OutDataTypeStr=single
  If : If  IfExpression=u1 > 180  ElseIfExpressions=u1 < -180
  If Action Subsystem : Subsystem  TreatAsAtomicUnit=on
  If Action Subsystem1 : Subsystem  TreatAsAtomicUnit=on
  If Action Subsystem2 : Subsystem  TreatAsAtomicUnit=on
  Merge : Merge  Inputs=3
  Out1 : Outport
  wires:
  In1/1 -> Add1/2, If Action Subsystem2/1(In1), Add/2, If/1
  If/1 -> If Action Subsystem/Action
  If/2 -> If Action Subsystem1/Action
  If/3 -> If Action Subsystem2/Action
  If Action Subsystem/1(Out1) -> Merge/1
  Constant/1 -> Add/1
  Add/1 -> If Action Subsystem/1(In1)
  If Action Subsystem1/1(Out1) -> Merge/2
  Constant1/1 -> Add1/1
  If Action Subsystem2/1(Out1) -> Merge/3
  Add1/1 -> If Action Subsystem1/1(In1)
  Merge/1 -> Out1/1

== system time/judgeLock/If Action Subsystem ==
  In1 : Inport
  Action Port : ActionPort
  Out1 : Outport
  wires:
  In1/1 -> Out1/1

== system time/judgeLock/If Action Subsystem1 ==
  In1 : Inport
  Action Port : ActionPort
  Out1 : Outport
  wires:
  In1/1 -> Out1/1

== system time/judgeLock1/If Action Subsystem ==
  In1 : Inport
  Action Port : ActionPort
  Out1 : Outport
  wires:
  In1/1 -> Out1/1

== system time/judgeLock1/If Action Subsystem1 ==
  In1 : Inport
  Action Port : ActionPort
  Out1 : Outport
  wires:
  In1/1 -> Out1/1

== system time/PWM/Subsystem/If Action Subsystem ==
  In1 : Inport
  Action Port : ActionPort
  Out1 : Outport
  wires:
  In1/1 -> Out1/1

== system time/PWM/Subsystem/If Action Subsystem1 ==
  In1 : Inport
  Action Port : ActionPort
  Out1 : Outport
  wires:
  In1/1 -> Out1/1

== system time/State Estimation and Complimentary Mixing/Complimentary Filter/Filter IC fixer ==
  FilterStart : Inport
  Normal Output : Inport  Port=2
  Constant : Constant
  IC : InitialCondition  Value=0
  Switch : Switch  Criteria=u2 ~= 0
  Out1 : Outport
  wires:
  Switch/1 -> Out1/1
  FilterStart/1 -> Switch/3
  IC/1 -> Switch/2
  Constant/1 -> IC/1
  Normal Output/1 -> Switch/1

== system time/State Estimation and Complimentary Mixing/Complimentary Filter/Filter IC fixer1 ==
  FilterStart : Inport
  Normal Output : Inport  Port=2
  Constant : Constant
  IC : InitialCondition  Value=0
  Switch : Switch  Criteria=u2 ~= 0
  Out1 : Outport
  wires:
  Switch/1 -> Out1/1
  FilterStart/1 -> Switch/3
  IC/1 -> Switch/2
  Constant/1 -> IC/1
  Normal Output/1 -> Switch/1

== system time/State Estimation and Complimentary Mixing/Complimentary Filter/Filter IC fixer2 ==
  FilterStart : Inport
  Normal Output : Inport  Port=2
  Constant : Constant
  IC : InitialCondition  Value=0
  Switch : Switch  Criteria=u2 ~= 0
  Out1 : Outport
  wires:
  Switch/1 -> Out1/1
  FilterStart/1 -> Switch/3
  IC/1 -> Switch/2
  Constant/1 -> IC/1
  Normal Output/1 -> Switch/1

== system time/State Estimation and Complimentary Mixing/Subsystem/Filter IC fixer1 ==
  FilterStart : Inport
  Normal Output : Inport  Port=2
  Constant : Constant
  IC : InitialCondition  Value=0
  Switch : Switch  Criteria=u2 ~= 0
  Out1 : Outport
  wires:
  Switch/1 -> Out1/1
  FilterStart/1 -> Switch/3
  IC/1 -> Switch/2
  Constant/1 -> IC/1
  Normal Output/1 -> Switch/1

== system time/State Estimation and Complimentary Mixing/Subsystem/Filter IC fixer2 ==
  FilterStart : Inport
  Normal Output : Inport  Port=2
  Constant : Constant
  IC : InitialCondition  Value=0
  Switch : Switch  Criteria=u2 ~= 0
  Out1 : Outport
  wires:
  Switch/1 -> Out1/1
  FilterStart/1 -> Switch/3
  IC/1 -> Switch/2
  Constant/1 -> IC/1
  Normal Output/1 -> Switch/1

== system time/State Estimation and Complimentary Mixing/Subsystem/Phi_dot composer ==
  note: H_Phi = [1,tan(The)*sin(Phi), tan(The)*cos(Phi);
      |          0,         cos(Phi),         -sin(Phi);
      |          0,sin(Phi)/cos(The),cos(Phi)/cos(The)];
      | Phidot = H_Phi*omb_bi; %% Units OK SI, this is the derivative of the Euler angles
  Phi : Inport
  Theta : Inport  Port=2
  P : Inport  Port=3
  Q : Inport  Port=4
  R : Inport  Port=5
  Product : Product  Inputs=3
  Product1 : Product  Inputs=3
  Sum : Sum  Inputs=+++
  Trigonometric Function : Trigonometry  Operator=tan
  Trigonometric Function1 : Trigonometry  Operator=sincos
  phiDot : Outport
  wires:
  Sum/1 -> phiDot/1
  Trigonometric Function/1 -> Product1/1, Product/1
  Product1/1 -> Sum/3
  Q/1 -> Product/3
  Trigonometric Function1/1 -> Product/2
  Phi/1 -> Trigonometric Function1/1
  Theta/1 -> Trigonometric Function/1
  P/1 -> Sum/1
  R/1 -> Product1/3
  Product/1 -> Sum/2
  Trigonometric Function1/2 -> Product1/2

== system time/State Estimation and Complimentary Mixing/Subsystem/Phi_dot composer1 ==
  note: H_Phi = [1,tan(The)*sin(Phi), tan(The)*cos(Phi);
      |          0,         cos(Phi),         -sin(Phi);
      |          0,sin(Phi)/cos(The),cos(Phi)/cos(The)];
      | Phidot = H_Phi*omb_bi; %% Units OK SI
  Phi : Inport
  Theta : Inport  Port=2
  Q : Inport  Port=3
  R : Inport  Port=4
  Divide : Product  Inputs=**/
  Divide1 : Product  Inputs=**/
  Sum : Sum  Inputs=|++
  Trigonometric Function : Trigonometry  Operator=sincos
  Trigonometric Function1 : Trigonometry  Operator=cos
  psiDot : Outport
  wires:
  Sum/1 -> psiDot/1
  Phi/1 -> Trigonometric Function/1
  Trigonometric Function/1 -> Divide/2
  Theta/1 -> Trigonometric Function1/1
  Divide/1 -> Sum/1
  Trigonometric Function1/1 -> Divide/3, Divide1/3
  Q/1 -> Divide/1
  R/1 -> Divide1/2
  Divide1/1 -> Sum/2
  Trigonometric Function/2 -> Divide1/1

== system time/State Estimation and Complimentary Mixing/Subsystem/Theta_dot composer1 ==
  note: H_Phi = [1,tan(The)*sin(Phi), tan(The)*cos(Phi);
      |          0,         cos(Phi),         -sin(Phi);
      |          0,sin(Phi)/cos(The),cos(Phi)/cos(The)];
      | Phidot = H_Phi*omb_bi; %% Units OK SI
  Phi : Inport
  Q : Inport  Port=2
  R : Inport  Port=3
  Product : Product
  Product1 : Product
  Scope : Scope  NumInputPorts=2
  Sum : Sum  Inputs=|++
  Trigonometric Function2 : Trigonometry  Operator=sincos
  Unary Minus : UnaryMinus
  thetaDot : Outport
  wires:
  Sum/1 -> thetaDot/1
  Phi/1 -> Trigonometric Function2/1
  Q/1 -> Product/2
  Product/1 -> Sum/1
  Trigonometric Function2/1 -> Scope/2, Unary Minus/1
  Unary Minus/1 -> Scope/1, Product1/1
  R/1 -> Product1/2
  Product1/1 -> Sum/2
  Trigonometric Function2/2 -> Product/1
